simulink library "pipelined_adc_library"  (R2019a)
settings: Solver=VariableStepAuto  StartTime=0.0  StopTime=10.0  RelTol=1e-3
libraries: $bdroot x1
settings Model: Creator=johan  LastModifiedBy=johan

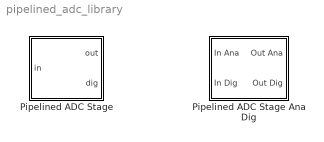
== system pipelined_adc_library ==
  Pipelined ADC Stage : Subsystem  mask{comp_offsets=[0, 0, 0, 0, 0, 0], sigma_noise=0, delta_G=0}
      mask prompts: comp_offsets "Comparator offsets"; sigma_noise "sigma noise"; delta_G "Delta G"
  Pipelined ADC Stage Ana Dig : Subsystem  mask{comp_offsets=[0, 0, 0, 0, 0, 0], sigma_noise=0, delta_G=0}
      mask prompts: comp_offsets "Comparator offsets"; sigma_noise "sigma noise"; delta_G "DeltaG"

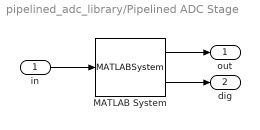
== system pipelined_adc_library/Pipelined ADC Stage ==
  in : Inport
  MATLAB System : MATLABSystem  System=pipelined_adc_stage  comp_offsets=comp_offsets  sigma_noise=sigma_noise  delta_G=delta_G  SimulateUsing=Code generation
      mask Type: pipelined_adc_stage
      mask Display:
      | disp('pipelined_adc_stage');
      | port_label('input',1,'u');
      | port_label('output',1,'y');
      | port_label('output',2,'q');
  out : Outport
  dig : Outport  Port=2
  wires:
  in/1 -> MATLAB System/1
  MATLAB System/1 -> out/1
  MATLAB System/2 -> dig/1

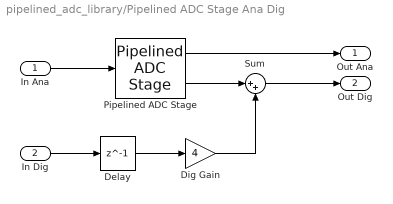
== system pipelined_adc_library/Pipelined ADC Stage Ana Dig ==
  In Ana : Inport
  In Dig : Inport  Port=2
  Delay : Delay  DelayLength=1  InitialCondition=0
  Dig Gain : Gain  Gain=4
  Pipelined ADC Stage : $bdroot/Pipelined ADC Stage  comp_offsets=comp_offsets  sigma_noise=sigma_noise  delta_G=delta_G
  Sum : Sum  Inputs=|++
  Out Ana : Outport
  Out Dig : Outport  Port=2
  wires:
  Delay/1 -> Dig Gain/1
  Pipelined ADC Stage/1 -> Out Ana/1
  Pipelined ADC Stage/2 -> Sum/1
  In Dig/1 -> Delay/1
  Dig Gain/1 -> Sum/2
  Sum/1 -> Out Dig/1
  In Ana/1 -> Pipelined ADC Stage/1
